simulink model "gm_rec_i2s"  (R2023b)
settings: Solver=VariableStepAuto  StartTime=0.0  StopTime=20  RelTol=1e-3
libraries: hdlsllib x2
(part 1 of 2)
settings Model: Creator=31651  LastModifiedBy=31651
settings DataIOCC: SignalLogging=off
settings OptimizationCC: BlockReduction=off  ConditionallyExecuteInputs=off  DefaultParameterBehavior=Inlined
settings DebuggingCC: AlgebraicLoopMsg=error  InheritedTsInSrcMsg=none
settings HardwareCC: ProdBitPerPointer=32  ProdBitPerSizeT=32  ProdBitPerPtrDiffT=32  ProdLargestAtomicFloat=None  ProdIntDivRoundTo=Undefined  ProdEndianess=Unspecified  ProdWordSize=32  ProdHWDeviceType=ASIC/FPGA->ASIC/FPGA  TargetBitPerPointer=64  TargetBitPerSizeT=64  TargetBitPerPtrDiffT=64  TargetLongLongMode=on  TargetIntDivRoundTo=Zero  TargetEndianess=LittleEndian  TargetWordSize=64  TargetHWDeviceType=Custom Processor->MATLAB Host Computer  ProdEqTarget=off

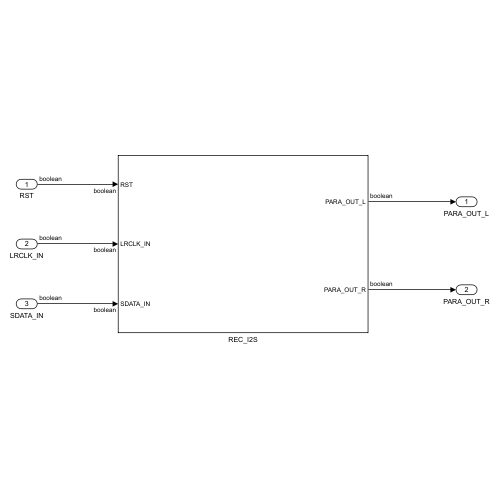
[thumbnail: Simulink's stored preview of the top-level diagram]
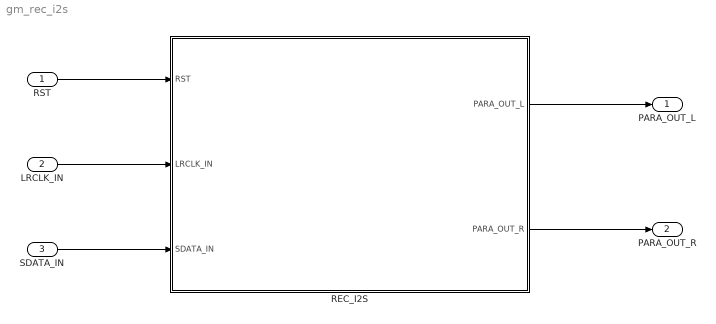
== system gm_rec_i2s ==
  RST : Inport  OutDataTypeStr=boolean  PortDimensions=1  SampleTime=1
  LRCLK_IN : Inport  Port=2  OutDataTypeStr=boolean  PortDimensions=1  SampleTime=1
  SDATA_IN : Inport  Port=3  OutDataTypeStr=boolean  PortDimensions=1  SampleTime=1
  REC_I2S : Subsystem
  PARA_OUT_L : Outport  SampleTime=1
  PARA_OUT_R : Outport  Port=2  SampleTime=1
  wires:
  RST/1 -> REC_I2S/1(RST)
  LRCLK_IN/1 -> REC_I2S/2(LRCLK_IN)
  SDATA_IN/1 -> REC_I2S/3(SDATA_IN)
  REC_I2S/1(PARA_OUT_L) -> PARA_OUT_L/1
  REC_I2S/2(PARA_OUT_R) -> PARA_OUT_R/1

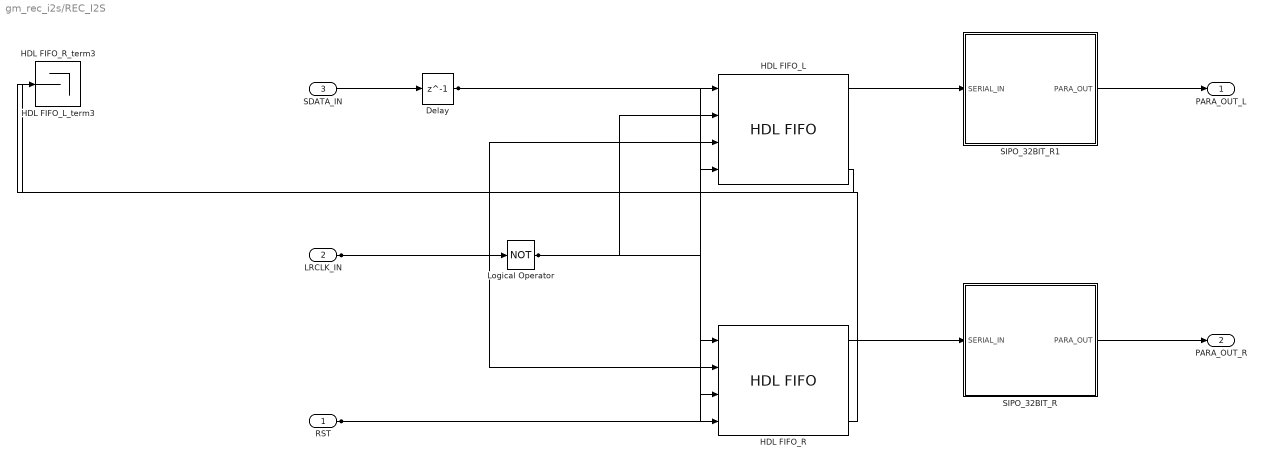
== system gm_rec_i2s/REC_I2S ==
  RST : Inport  OutDataTypeStr=boolean  PortDimensions=1  SampleTime=1
  LRCLK_IN : Inport  Port=2  OutDataTypeStr=boolean  PortDimensions=1  SampleTime=1
  SDATA_IN : Inport  Port=3  OutDataTypeStr=boolean  PortDimensions=1  SampleTime=1
  Delay : Delay  DelayLength=1  InitialCondition=0  SampleTime=1
  HDL FIFO_L : hdlsllib/HDL RAMs/HDL FIFO  fifo_size=32  mode=Classic  ratio=1  push_msg=Warning  pop_msg=Warning  show_empty=on  show_full=on  show_num=on  LabelModeActiveChoice_Mode=Classic  rst_port=on
  HDL FIFO_L_term3 : Terminator
  HDL FIFO_R : hdlsllib/HDL RAMs/HDL FIFO  fifo_size=32  mode=Classic  ratio=1  push_msg=Warning  pop_msg=Warning  show_empty=on  show_full=on  show_num=on  LabelModeActiveChoice_Mode=Classic  rst_port=on
  HDL FIFO_R_term3 : Terminator
  Logical Operator : Logic  Operator=NOT  AllPortsSameDT=off  OutDataTypeStr=boolean
  SIPO_32BIT_R : Subsystem
  SIPO_32BIT_R1 : Subsystem
  PARA_OUT_L : Outport  OutDataTypeStr=boolean  SampleTime=1
  PARA_OUT_R : Outport  Port=2  OutDataTypeStr=boolean  SampleTime=1
  wires:
  RST/1 -> HDL FIFO_R/4, HDL FIFO_L/4
  LRCLK_IN/1 -> Logical Operator/1, HDL FIFO_R/2, HDL FIFO_L/3
  SDATA_IN/1 -> Delay/1
  Delay/1 -> HDL FIFO_R/1, HDL FIFO_L/1
  HDL FIFO_L/1 -> SIPO_32BIT_R1/1(SERIAL_IN)
  HDL FIFO_L/4 -> HDL FIFO_L_term3/1
  HDL FIFO_R/1 -> SIPO_32BIT_R/1(SERIAL_IN)
  HDL FIFO_R/4 -> HDL FIFO_R_term3/1
  Logical Operator/1 -> HDL FIFO_R/3, HDL FIFO_L/2
  SIPO_32BIT_R/1(PARA_OUT) -> PARA_OUT_R/1
  SIPO_32BIT_R1/1(PARA_OUT) -> PARA_OUT_L/1

== system gm_rec_i2s/REC_I2S/SIPO_32BIT_R ==
  SERIAL_IN : Inport  OutDataTypeStr=boolean  PortDimensions=1  SampleTime=1
  Subsystem : Subsystem
  PARA_OUT : Outport  OutDataTypeStr=boolean  SampleTime=1  VectorParamsAs1DForOutWhenUnconnected=off
  wires:
  SERIAL_IN/1 -> Subsystem/1(SERIAL_IN)
  Subsystem/1(PARA_OUT_32BIT) -> PARA_OUT/1

== system gm_rec_i2s/REC_I2S/SIPO_32BIT_R1 ==
  SERIAL_IN : Inport  OutDataTypeStr=boolean  PortDimensions=1  SampleTime=1
  Subsystem : Subsystem
  PARA_OUT : Outport  OutDataTypeStr=boolean  SampleTime=1  VectorParamsAs1DForOutWhenUnconnected=off
  wires:
  SERIAL_IN/1 -> Subsystem/1(SERIAL_IN)
  Subsystem/1(PARA_OUT_32BIT) -> PARA_OUT/1

== system gm_rec_i2s/REC_I2S/SIPO_32BIT_R/Subsystem ==
  SERIAL_IN : Inport  OutDataTypeStr=boolean  PortDimensions=1  SampleTime=1
  SIPO_16BIT : Subsystem
  SIPO_16BIT1 : Subsystem
  Vector Concatenate : Concatenate
  PARA_OUT_32BIT : Outport  SampleTime=1
  wires:
  SERIAL_IN/1 -> SIPO_16BIT/1(SERIAL_IN)
  SIPO_16BIT/1(PARA_OUT) -> Vector Concatenate/2
  SIPO_16BIT/2(SERIAL_OUT) -> SIPO_16BIT1/1(SERIAL_IN)
  SIPO_16BIT1/1(PARA_OUT) -> Vector Concatenate/1
  Vector Concatenate/1 -> PARA_OUT_32BIT/1

== system gm_rec_i2s/REC_I2S/SIPO_32BIT_R1/Subsystem ==
  SERIAL_IN : Inport  OutDataTypeStr=boolean  PortDimensions=1  SampleTime=1
  SIPO_16BIT : Subsystem
  SIPO_16BIT1 : Subsystem
  Vector Concatenate : Concatenate
  PARA_OUT_32BIT : Outport  SampleTime=1
  wires:
  SERIAL_IN/1 -> SIPO_16BIT/1(SERIAL_IN)
  SIPO_16BIT/1(PARA_OUT) -> Vector Concatenate/2
  SIPO_16BIT/2(SERIAL_OUT) -> SIPO_16BIT1/1(SERIAL_IN)
  SIPO_16BIT1/1(PARA_OUT) -> Vector Concatenate/1
  Vector Concatenate/1 -> PARA_OUT_32BIT/1

== system gm_rec_i2s/REC_I2S/SIPO_32BIT_R/Subsystem/SIPO_16BIT ==
  SERIAL_IN : Inport  OutDataTypeStr=boolean  PortDimensions=1  SampleTime=1
  SIPO_8BIT : Subsystem
  SIPO_8BIT1 : Subsystem
  Vector Concatenate : Concatenate
  PARA_OUT : Outport  OutDataTypeStr=boolean  SampleTime=1  VectorParamsAs1DForOutWhenUnconnected=off
  SERIAL_OUT : Outport  Port=2  OutDataTypeStr=boolean  SampleTime=1  VectorParamsAs1DForOutWhenUnconnected=off
  wires:
  SERIAL_IN/1 -> SIPO_8BIT/1(SERIAL_IN)
  SIPO_8BIT/1(PARA_OUT) -> Vector Concatenate/2
  SIPO_8BIT/2(SERIAL_OUT) -> SIPO_8BIT1/1(SERIAL_IN)
  SIPO_8BIT1/1(PARA_OUT) -> Vector Concatenate/1
  SIPO_8BIT1/2(SERIAL_OUT) -> SERIAL_OUT/1
  Vector Concatenate/1 -> PARA_OUT/1

== system gm_rec_i2s/REC_I2S/SIPO_32BIT_R/Subsystem/SIPO_16BIT1 ==
  SERIAL_IN : Inport  OutDataTypeStr=boolean  PortDimensions=1  SampleTime=1
  SIPO_8BIT : Subsystem
  SIPO_8BIT1 : Subsystem
  Vector Concatenate : Concatenate
  PARA_OUT : Outport  OutDataTypeStr=boolean  SampleTime=1  VectorParamsAs1DForOutWhenUnconnected=off
  wires:
  SERIAL_IN/1 -> SIPO_8BIT/1(SERIAL_IN)
  SIPO_8BIT/1(PARA_OUT) -> Vector Concatenate/2
  SIPO_8BIT/2(SERIAL_OUT) -> SIPO_8BIT1/1(SERIAL_IN)
  SIPO_8BIT1/1(PARA_OUT) -> Vector Concatenate/1
  Vector Concatenate/1 -> PARA_OUT/1

== system gm_rec_i2s/REC_I2S/SIPO_32BIT_R1/Subsystem/SIPO_16BIT ==
  SERIAL_IN : Inport  OutDataTypeStr=boolean  PortDimensions=1  SampleTime=1
  SIPO_8BIT : Subsystem
  SIPO_8BIT1 : Subsystem
  Vector Concatenate : Concatenate
  PARA_OUT : Outport  OutDataTypeStr=boolean  SampleTime=1  VectorParamsAs1DForOutWhenUnconnected=off
  SERIAL_OUT : Outport  Port=2  OutDataTypeStr=boolean  SampleTime=1  VectorParamsAs1DForOutWhenUnconnected=off
  wires:
  SERIAL_IN/1 -> SIPO_8BIT/1(SERIAL_IN)
  SIPO_8BIT/1(PARA_OUT) -> Vector Concatenate/2
  SIPO_8BIT/2(SERIAL_OUT) -> SIPO_8BIT1/1(SERIAL_IN)
  SIPO_8BIT1/1(PARA_OUT) -> Vector Concatenate/1
  SIPO_8BIT1/2(SERIAL_OUT) -> SERIAL_OUT/1
  Vector Concatenate/1 -> PARA_OUT/1

== system gm_rec_i2s/REC_I2S/SIPO_32BIT_R1/Subsystem/SIPO_16BIT1 ==
  SERIAL_IN : Inport  OutDataTypeStr=boolean  PortDimensions=1  SampleTime=1
  SIPO_8BIT : Subsystem
  SIPO_8BIT1 : Subsystem
  Vector Concatenate : Concatenate
  PARA_OUT : Outport  OutDataTypeStr=boolean  SampleTime=1  VectorParamsAs1DForOutWhenUnconnected=off
  wires:
  SERIAL_IN/1 -> SIPO_8BIT/1(SERIAL_IN)
  SIPO_8BIT/1(PARA_OUT) -> Vector Concatenate/2
  SIPO_8BIT/2(SERIAL_OUT) -> SIPO_8BIT1/1(SERIAL_IN)
  SIPO_8BIT1/1(PARA_OUT) -> Vector Concatenate/1
  Vector Concatenate/1 -> PARA_OUT/1

== system gm_rec_i2s/REC_I2S/SIPO_32BIT_R/Subsystem/SIPO_16BIT/SIPO_8BIT ==
  SERIAL_IN : Inport  OutDataTypeStr=boolean  PortDimensions=1  SampleTime=1
  SIPO_4BIT : Subsystem
  SIPO_4BIT1 : Subsystem
  Vector Concatenate : Concatenate
  PARA_OUT : Outport  SampleTime=1  VectorParamsAs1DForOutWhenUnconnected=off
  SERIAL_OUT : Outport  Port=2  SampleTime=1  VectorParamsAs1DForOutWhenUnconnected=off
  wires:
  SERIAL_IN/1 -> SIPO_4BIT/1(SERIAL_IN)
  SIPO_4BIT/1(PARA_OUT) -> Vector Concatenate/2
  SIPO_4BIT/2(SERIAL_OUT) -> SIPO_4BIT1/1(SERIAL_IN)
  SIPO_4BIT1/1(PARA_OUT) -> Vector Concatenate/1
  SIPO_4BIT1/2(SERIAL_OUT) -> SERIAL_OUT/1
  Vector Concatenate/1 -> PARA_OUT/1

== system gm_rec_i2s/REC_I2S/SIPO_32BIT_R/Subsystem/SIPO_16BIT/SIPO_8BIT1 ==
  SERIAL_IN : Inport  OutDataTypeStr=boolean  PortDimensions=1  SampleTime=1
  SIPO_4BIT : Subsystem
  SIPO_4BIT1 : Subsystem
  Vector Concatenate : Concatenate
  PARA_OUT : Outport  SampleTime=1  VectorParamsAs1DForOutWhenUnconnected=off
  SERIAL_OUT : Outport  Port=2  SampleTime=1  VectorParamsAs1DForOutWhenUnconnected=off
  wires:
  SERIAL_IN/1 -> SIPO_4BIT/1(SERIAL_IN)
  SIPO_4BIT/1(PARA_OUT) -> Vector Concatenate/2
  SIPO_4BIT/2(SERIAL_OUT) -> SIPO_4BIT1/1(SERIAL_IN)
  SIPO_4BIT1/1(PARA_OUT) -> Vector Concatenate/1
  SIPO_4BIT1/2(SERIAL_OUT) -> SERIAL_OUT/1
  Vector Concatenate/1 -> PARA_OUT/1

== system gm_rec_i2s/REC_I2S/SIPO_32BIT_R/Subsystem/SIPO_16BIT1/SIPO_8BIT ==
  SERIAL_IN : Inport  OutDataTypeStr=boolean  PortDimensions=1  SampleTime=1
  SIPO_4BIT : Subsystem
  SIPO_4BIT1 : Subsystem
  Vector Concatenate : Concatenate
  PARA_OUT : Outport  SampleTime=1  VectorParamsAs1DForOutWhenUnconnected=off
  SERIAL_OUT : Outport  Port=2  SampleTime=1  VectorParamsAs1DForOutWhenUnconnected=off
  wires:
  SERIAL_IN/1 -> SIPO_4BIT/1(SERIAL_IN)
  SIPO_4BIT/1(PARA_OUT) -> Vector Concatenate/2
  SIPO_4BIT/2(SERIAL_OUT) -> SIPO_4BIT1/1(SERIAL_IN)
  SIPO_4BIT1/1(PARA_OUT) -> Vector Concatenate/1
  SIPO_4BIT1/2(SERIAL_OUT) -> SERIAL_OUT/1
  Vector Concatenate/1 -> PARA_OUT/1

== system gm_rec_i2s/REC_I2S/SIPO_32BIT_R/Subsystem/SIPO_16BIT1/SIPO_8BIT1 ==
  SERIAL_IN : Inport  OutDataTypeStr=boolean  PortDimensions=1  SampleTime=1
  SIPO_4BIT : Subsystem
  SIPO_4BIT1 : Subsystem
  Vector Concatenate : Concatenate
  PARA_OUT : Outport  SampleTime=1  VectorParamsAs1DForOutWhenUnconnected=off
  wires:
  SERIAL_IN/1 -> SIPO_4BIT/1(SERIAL_IN)
  SIPO_4BIT/1(PARA_OUT) -> Vector Concatenate/2
  SIPO_4BIT/2(SERIAL_OUT) -> SIPO_4BIT1/1(SERIAL_IN)
  SIPO_4BIT1/1(PARA_OUT) -> Vector Concatenate/1
  Vector Concatenate/1 -> PARA_OUT/1

== system gm_rec_i2s/REC_I2S/SIPO_32BIT_R1/Subsystem/SIPO_16BIT/SIPO_8BIT ==
  SERIAL_IN : Inport  OutDataTypeStr=boolean  PortDimensions=1  SampleTime=1
  SIPO_4BIT : Subsystem
  SIPO_4BIT1 : Subsystem
  Vector Concatenate : Concatenate
  PARA_OUT : Outport  SampleTime=1  VectorParamsAs1DForOutWhenUnconnected=off
  SERIAL_OUT : Outport  Port=2  SampleTime=1  VectorParamsAs1DForOutWhenUnconnected=off
  wires:
  SERIAL_IN/1 -> SIPO_4BIT/1(SERIAL_IN)
  SIPO_4BIT/1(PARA_OUT) -> Vector Concatenate/2
  SIPO_4BIT/2(SERIAL_OUT) -> SIPO_4BIT1/1(SERIAL_IN)
  SIPO_4BIT1/1(PARA_OUT) -> Vector Concatenate/1
  SIPO_4BIT1/2(SERIAL_OUT) -> SERIAL_OUT/1
  Vector Concatenate/1 -> PARA_OUT/1

== system gm_rec_i2s/REC_I2S/SIPO_32BIT_R1/Subsystem/SIPO_16BIT/SIPO_8BIT1 ==
  SERIAL_IN : Inport  OutDataTypeStr=boolean  PortDimensions=1  SampleTime=1
  SIPO_4BIT : Subsystem
  SIPO_4BIT1 : Subsystem
  Vector Concatenate : Concatenate
  PARA_OUT : Outport  SampleTime=1  VectorParamsAs1DForOutWhenUnconnected=off
  SERIAL_OUT : Outport  Port=2  SampleTime=1  VectorParamsAs1DForOutWhenUnconnected=off
  wires:
  SERIAL_IN/1 -> SIPO_4BIT/1(SERIAL_IN)
  SIPO_4BIT/1(PARA_OUT) -> Vector Concatenate/2
  SIPO_4BIT/2(SERIAL_OUT) -> SIPO_4BIT1/1(SERIAL_IN)
  SIPO_4BIT1/1(PARA_OUT) -> Vector Concatenate/1
  SIPO_4BIT1/2(SERIAL_OUT) -> SERIAL_OUT/1
  Vector Concatenate/1 -> PARA_OUT/1

== system gm_rec_i2s/REC_I2S/SIPO_32BIT_R1/Subsystem/SIPO_16BIT1/SIPO_8BIT ==
  SERIAL_IN : Inport  OutDataTypeStr=boolean  PortDimensions=1  SampleTime=1
  SIPO_4BIT : Subsystem
  SIPO_4BIT1 : Subsystem
  Vector Concatenate : Concatenate
  PARA_OUT : Outport  SampleTime=1  VectorParamsAs1DForOutWhenUnconnected=off
  SERIAL_OUT : Outport  Port=2  SampleTime=1  VectorParamsAs1DForOutWhenUnconnected=off
  wires:
  SERIAL_IN/1 -> SIPO_4BIT/1(SERIAL_IN)
  SIPO_4BIT/1(PARA_OUT) -> Vector Concatenate/2
  SIPO_4BIT/2(SERIAL_OUT) -> SIPO_4BIT1/1(SERIAL_IN)
  SIPO_4BIT1/1(PARA_OUT) -> Vector Concatenate/1
  SIPO_4BIT1/2(SERIAL_OUT) -> SERIAL_OUT/1
  Vector Concatenate/1 -> PARA_OUT/1

== system gm_rec_i2s/REC_I2S/SIPO_32BIT_R1/Subsystem/SIPO_16BIT1/SIPO_8BIT1 ==
  SERIAL_IN : Inport  OutDataTypeStr=boolean  PortDimensions=1  SampleTime=1
  SIPO_4BIT : Subsystem
  SIPO_4BIT1 : Subsystem
  Vector Concatenate : Concatenate
  PARA_OUT : Outport  SampleTime=1  VectorParamsAs1DForOutWhenUnconnected=off
  wires:
  SERIAL_IN/1 -> SIPO_4BIT/1(SERIAL_IN)
  SIPO_4BIT/1(PARA_OUT) -> Vector Concatenate/2
  SIPO_4BIT/2(SERIAL_OUT) -> SIPO_4BIT1/1(SERIAL_IN)
  SIPO_4BIT1/1(PARA_OUT) -> Vector Concatenate/1
  Vector Concatenate/1 -> PARA_OUT/1

== system gm_rec_i2s/REC_I2S/SIPO_32BIT_R/Subsystem/SIPO_16BIT/SIPO_8BIT/SIPO_4BIT ==
  SERIAL_IN : Inport  OutDataTypeStr=boolean  PortDimensions=1  SampleTime=1
  2BIT_SIPO : Subsystem
  2BIT_SIPO1 : Subsystem
  Vector Concatenate : Concatenate
  PARA_OUT : Outport  SampleTime=1  VectorParamsAs1DForOutWhenUnconnected=off
  SERIAL_OUT : Outport  Port=2  SampleTime=1  VectorParamsAs1DForOutWhenUnconnected=off
  wires:
  SERIAL_IN/1 -> 2BIT_SIPO/1(SERIAL_IN)
  2BIT_SIPO/1(PARA_OUT) -> Vector Concatenate/2
  2BIT_SIPO/2(SERIAL_OUT) -> 2BIT_SIPO1/1(SERIAL_IN)
  2BIT_SIPO1/1(PARA_OUT) -> Vector Concatenate/1
  2BIT_SIPO1/2(SERIAL_OUT) -> SERIAL_OUT/1
  Vector Concatenate/1 -> PARA_OUT/1

== system gm_rec_i2s/REC_I2S/SIPO_32BIT_R/Subsystem/SIPO_16BIT/SIPO_8BIT/SIPO_4BIT1 ==
  SERIAL_IN : Inport  OutDataTypeStr=boolean  PortDimensions=1  SampleTime=1
  2BIT_SIPO : Subsystem
  2BIT_SIPO1 : Subsystem
  Vector Concatenate : Concatenate
  PARA_OUT : Outport  SampleTime=1  VectorParamsAs1DForOutWhenUnconnected=off
  SERIAL_OUT : Outport  Port=2  SampleTime=1  VectorParamsAs1DForOutWhenUnconnected=off
  wires:
  SERIAL_IN/1 -> 2BIT_SIPO/1(SERIAL_IN)
  2BIT_SIPO/1(PARA_OUT) -> Vector Concatenate/2
  2BIT_SIPO/2(SERIAL_OUT) -> 2BIT_SIPO1/1(SERIAL_IN)
  2BIT_SIPO1/1(PARA_OUT) -> Vector Concatenate/1
  2BIT_SIPO1/2(SERIAL_OUT) -> SERIAL_OUT/1
  Vector Concatenate/1 -> PARA_OUT/1

== system gm_rec_i2s/REC_I2S/SIPO_32BIT_R/Subsystem/SIPO_16BIT/SIPO_8BIT1/SIPO_4BIT ==
  SERIAL_IN : Inport  OutDataTypeStr=boolean  PortDimensions=1  SampleTime=1
  2BIT_SIPO : Subsystem
  2BIT_SIPO1 : Subsystem
  Vector Concatenate : Concatenate
  PARA_OUT : Outport  SampleTime=1  VectorParamsAs1DForOutWhenUnconnected=off
  SERIAL_OUT : Outport  Port=2  SampleTime=1  VectorParamsAs1DForOutWhenUnconnected=off
  wires:
  SERIAL_IN/1 -> 2BIT_SIPO/1(SERIAL_IN)
  2BIT_SIPO/1(PARA_OUT) -> Vector Concatenate/2
  2BIT_SIPO/2(SERIAL_OUT) -> 2BIT_SIPO1/1(SERIAL_IN)
  2BIT_SIPO1/1(PARA_OUT) -> Vector Concatenate/1
  2BIT_SIPO1/2(SERIAL_OUT) -> SERIAL_OUT/1
  Vector Concatenate/1 -> PARA_OUT/1

== system gm_rec_i2s/REC_I2S/SIPO_32BIT_R/Subsystem/SIPO_16BIT/SIPO_8BIT1/SIPO_4BIT1 ==
  SERIAL_IN : Inport  OutDataTypeStr=boolean  PortDimensions=1  SampleTime=1
  2BIT_SIPO : Subsystem
  2BIT_SIPO1 : Subsystem
  Vector Concatenate : Concatenate
  PARA_OUT : Outport  SampleTime=1  VectorParamsAs1DForOutWhenUnconnected=off
  SERIAL_OUT : Outport  Port=2  SampleTime=1  VectorParamsAs1DForOutWhenUnconnected=off
  wires:
  SERIAL_IN/1 -> 2BIT_SIPO/1(SERIAL_IN)
  2BIT_SIPO/1(PARA_OUT) -> Vector Concatenate/2
  2BIT_SIPO/2(SERIAL_OUT) -> 2BIT_SIPO1/1(SERIAL_IN)
  2BIT_SIPO1/1(PARA_OUT) -> Vector Concatenate/1
  2BIT_SIPO1/2(SERIAL_OUT) -> SERIAL_OUT/1
  Vector Concatenate/1 -> PARA_OUT/1

== system gm_rec_i2s/REC_I2S/SIPO_32BIT_R/Subsystem/SIPO_16BIT1/SIPO_8BIT/SIPO_4BIT ==
  SERIAL_IN : Inport  OutDataTypeStr=boolean  PortDimensions=1  SampleTime=1
  2BIT_SIPO : Subsystem
  2BIT_SIPO1 : Subsystem
  Vector Concatenate : Concatenate
  PARA_OUT : Outport  SampleTime=1  VectorParamsAs1DForOutWhenUnconnected=off
  SERIAL_OUT : Outport  Port=2  SampleTime=1  VectorParamsAs1DForOutWhenUnconnected=off
  wires:
  SERIAL_IN/1 -> 2BIT_SIPO/1(SERIAL_IN)
  2BIT_SIPO/1(PARA_OUT) -> Vector Concatenate/2
  2BIT_SIPO/2(SERIAL_OUT) -> 2BIT_SIPO1/1(SERIAL_IN)
  2BIT_SIPO1/1(PARA_OUT) -> Vector Concatenate/1
  2BIT_SIPO1/2(SERIAL_OUT) -> SERIAL_OUT/1
  Vector Concatenate/1 -> PARA_OUT/1

== system gm_rec_i2s/REC_I2S/SIPO_32BIT_R/Subsystem/SIPO_16BIT1/SIPO_8BIT/SIPO_4BIT1 ==
  SERIAL_IN : Inport  OutDataTypeStr=boolean  PortDimensions=1  SampleTime=1
  2BIT_SIPO : Subsystem
  2BIT_SIPO1 : Subsystem
  Vector Concatenate : Concatenate
  PARA_OUT : Outport  SampleTime=1  VectorParamsAs1DForOutWhenUnconnected=off
  SERIAL_OUT : Outport  Port=2  SampleTime=1  VectorParamsAs1DForOutWhenUnconnected=off
  wires:
  SERIAL_IN/1 -> 2BIT_SIPO/1(SERIAL_IN)
  2BIT_SIPO/1(PARA_OUT) -> Vector Concatenate/2
  2BIT_SIPO/2(SERIAL_OUT) -> 2BIT_SIPO1/1(SERIAL_IN)
  2BIT_SIPO1/1(PARA_OUT) -> Vector Concatenate/1
  2BIT_SIPO1/2(SERIAL_OUT) -> SERIAL_OUT/1
  Vector Concatenate/1 -> PARA_OUT/1

== system gm_rec_i2s/REC_I2S/SIPO_32BIT_R/Subsystem/SIPO_16BIT1/SIPO_8BIT1/SIPO_4BIT ==
  SERIAL_IN : Inport  OutDataTypeStr=boolean  PortDimensions=1  SampleTime=1
  2BIT_SIPO : Subsystem
  2BIT_SIPO1 : Subsystem
  Vector Concatenate : Concatenate
  PARA_OUT : Outport  SampleTime=1  VectorParamsAs1DForOutWhenUnconnected=off
  SERIAL_OUT : Outport  Port=2  SampleTime=1  VectorParamsAs1DForOutWhenUnconnected=off
  wires:
  SERIAL_IN/1 -> 2BIT_SIPO/1(SERIAL_IN)
  2BIT_SIPO/1(PARA_OUT) -> Vector Concatenate/2
  2BIT_SIPO/2(SERIAL_OUT) -> 2BIT_SIPO1/1(SERIAL_IN)
  2BIT_SIPO1/1(PARA_OUT) -> Vector Concatenate/1
  2BIT_SIPO1/2(SERIAL_OUT) -> SERIAL_OUT/1
  Vector Concatenate/1 -> PARA_OUT/1

== system gm_rec_i2s/REC_I2S/SIPO_32BIT_R/Subsystem/SIPO_16BIT1/SIPO_8BIT1/SIPO_4BIT1 ==
  SERIAL_IN : Inport  OutDataTypeStr=boolean  PortDimensions=1  SampleTime=1
  2BIT_SIPO : Subsystem
  2BIT_SIPO1 : Subsystem
  Vector Concatenate : Concatenate
  PARA_OUT : Outport  SampleTime=1  VectorParamsAs1DForOutWhenUnconnected=off
  wires:
  SERIAL_IN/1 -> 2BIT_SIPO/1(SERIAL_IN)
  2BIT_SIPO/1(PARA_OUT) -> Vector Concatenate/2
  2BIT_SIPO/2(SERIAL_OUT) -> 2BIT_SIPO1/1(SERIAL_IN)
  2BIT_SIPO1/1(PARA_OUT) -> Vector Concatenate/1
  Vector Concatenate/1 -> PARA_OUT/1

== system gm_rec_i2s/REC_I2S/SIPO_32BIT_R1/Subsystem/SIPO_16BIT/SIPO_8BIT/SIPO_4BIT ==
  SERIAL_IN : Inport  OutDataTypeStr=boolean  PortDimensions=1  SampleTime=1
  2BIT_SIPO : Subsystem
  2BIT_SIPO1 : Subsystem
  Vector Concatenate : Concatenate
  PARA_OUT : Outport  SampleTime=1  VectorParamsAs1DForOutWhenUnconnected=off
  SERIAL_OUT : Outport  Port=2  SampleTime=1  VectorParamsAs1DForOutWhenUnconnected=off
  wires:
  SERIAL_IN/1 -> 2BIT_SIPO/1(SERIAL_IN)
  2BIT_SIPO/1(PARA_OUT) -> Vector Concatenate/2
  2BIT_SIPO/2(SERIAL_OUT) -> 2BIT_SIPO1/1(SERIAL_IN)
  2BIT_SIPO1/1(PARA_OUT) -> Vector Concatenate/1
  2BIT_SIPO1/2(SERIAL_OUT) -> SERIAL_OUT/1
  Vector Concatenate/1 -> PARA_OUT/1

== system gm_rec_i2s/REC_I2S/SIPO_32BIT_R1/Subsystem/SIPO_16BIT/SIPO_8BIT/SIPO_4BIT1 ==
  SERIAL_IN : Inport  OutDataTypeStr=boolean  PortDimensions=1  SampleTime=1
  2BIT_SIPO : Subsystem
  2BIT_SIPO1 : Subsystem
  Vector Concatenate : Concatenate
  PARA_OUT : Outport  SampleTime=1  VectorParamsAs1DForOutWhenUnconnected=off
  SERIAL_OUT : Outport  Port=2  SampleTime=1  VectorParamsAs1DForOutWhenUnconnected=off
  wires:
  SERIAL_IN/1 -> 2BIT_SIPO/1(SERIAL_IN)
  2BIT_SIPO/1(PARA_OUT) -> Vector Concatenate/2
  2BIT_SIPO/2(SERIAL_OUT) -> 2BIT_SIPO1/1(SERIAL_IN)
  2BIT_SIPO1/1(PARA_OUT) -> Vector Concatenate/1
  2BIT_SIPO1/2(SERIAL_OUT) -> SERIAL_OUT/1
  Vector Concatenate/1 -> PARA_OUT/1

== system gm_rec_i2s/REC_I2S/SIPO_32BIT_R1/Subsystem/SIPO_16BIT/SIPO_8BIT1/SIPO_4BIT ==
  SERIAL_IN : Inport  OutDataTypeStr=boolean  PortDimensions=1  SampleTime=1
  2BIT_SIPO : Subsystem
  2BIT_SIPO1 : Subsystem
  Vector Concatenate : Concatenate
  PARA_OUT : Outport  SampleTime=1  VectorParamsAs1DForOutWhenUnconnected=off
  SERIAL_OUT : Outport  Port=2  SampleTime=1  VectorParamsAs1DForOutWhenUnconnected=off
  wires:
  SERIAL_IN/1 -> 2BIT_SIPO/1(SERIAL_IN)
  2BIT_SIPO/1(PARA_OUT) -> Vector Concatenate/2
  2BIT_SIPO/2(SERIAL_OUT) -> 2BIT_SIPO1/1(SERIAL_IN)
  2BIT_SIPO1/1(PARA_OUT) -> Vector Concatenate/1
  2BIT_SIPO1/2(SERIAL_OUT) -> SERIAL_OUT/1
  Vector Concatenate/1 -> PARA_OUT/1

== system gm_rec_i2s/REC_I2S/SIPO_32BIT_R1/Subsystem/SIPO_16BIT/SIPO_8BIT1/SIPO_4BIT1 ==
  SERIAL_IN : Inport  OutDataTypeStr=boolean  PortDimensions=1  SampleTime=1
  2BIT_SIPO : Subsystem
  2BIT_SIPO1 : Subsystem
  Vector Concatenate : Concatenate
  PARA_OUT : Outport  SampleTime=1  VectorParamsAs1DForOutWhenUnconnected=off
  SERIAL_OUT : Outport  Port=2  SampleTime=1  VectorParamsAs1DForOutWhenUnconnected=off
  wires:
  SERIAL_IN/1 -> 2BIT_SIPO/1(SERIAL_IN)
  2BIT_SIPO/1(PARA_OUT) -> Vector Concatenate/2
  2BIT_SIPO/2(SERIAL_OUT) -> 2BIT_SIPO1/1(SERIAL_IN)
  2BIT_SIPO1/1(PARA_OUT) -> Vector Concatenate/1
  2BIT_SIPO1/2(SERIAL_OUT) -> SERIAL_OUT/1
  Vector Concatenate/1 -> PARA_OUT/1

== system gm_rec_i2s/REC_I2S/SIPO_32BIT_R1/Subsystem/SIPO_16BIT1/SIPO_8BIT/SIPO_4BIT ==
  SERIAL_IN : Inport  OutDataTypeStr=boolean  PortDimensions=1  SampleTime=1
  2BIT_SIPO : Subsystem
  2BIT_SIPO1 : Subsystem
  Vector Concatenate : Concatenate
  PARA_OUT : Outport  SampleTime=1  VectorParamsAs1DForOutWhenUnconnected=off
  SERIAL_OUT : Outport  Port=2  SampleTime=1  VectorParamsAs1DForOutWhenUnconnected=off
  wires:
  SERIAL_IN/1 -> 2BIT_SIPO/1(SERIAL_IN)
  2BIT_SIPO/1(PARA_OUT) -> Vector Concatenate/2
  2BIT_SIPO/2(SERIAL_OUT) -> 2BIT_SIPO1/1(SERIAL_IN)
  2BIT_SIPO1/1(PARA_OUT) -> Vector Concatenate/1
  2BIT_SIPO1/2(SERIAL_OUT) -> SERIAL_OUT/1
  Vector Concatenate/1 -> PARA_OUT/1

== system gm_rec_i2s/REC_I2S/SIPO_32BIT_R1/Subsystem/SIPO_16BIT1/SIPO_8BIT/SIPO_4BIT1 ==
  SERIAL_IN : Inport  OutDataTypeStr=boolean  PortDimensions=1  SampleTime=1
  2BIT_SIPO : Subsystem
  2BIT_SIPO1 : Subsystem
  Vector Concatenate : Concatenate
  PARA_OUT : Outport  SampleTime=1  VectorParamsAs1DForOutWhenUnconnected=off
  SERIAL_OUT : Outport  Port=2  SampleTime=1  VectorParamsAs1DForOutWhenUnconnected=off
  wires:
  SERIAL_IN/1 -> 2BIT_SIPO/1(SERIAL_IN)
  2BIT_SIPO/1(PARA_OUT) -> Vector Concatenate/2
  2BIT_SIPO/2(SERIAL_OUT) -> 2BIT_SIPO1/1(SERIAL_IN)
  2BIT_SIPO1/1(PARA_OUT) -> Vector Concatenate/1
  2BIT_SIPO1/2(SERIAL_OUT) -> SERIAL_OUT/1
  Vector Concatenate/1 -> PARA_OUT/1

== system gm_rec_i2s/REC_I2S/SIPO_32BIT_R1/Subsystem/SIPO_16BIT1/SIPO_8BIT1/SIPO_4BIT ==
  SERIAL_IN : Inport  OutDataTypeStr=boolean  PortDimensions=1  SampleTime=1
  2BIT_SIPO : Subsystem
  2BIT_SIPO1 : Subsystem
  Vector Concatenate : Concatenate
  PARA_OUT : Outport  SampleTime=1  VectorParamsAs1DForOutWhenUnconnected=off
  SERIAL_OUT : Outport  Port=2  SampleTime=1  VectorParamsAs1DForOutWhenUnconnected=off
  wires:
  SERIAL_IN/1 -> 2BIT_SIPO/1(SERIAL_IN)
  2BIT_SIPO/1(PARA_OUT) -> Vector Concatenate/2
  2BIT_SIPO/2(SERIAL_OUT) -> 2BIT_SIPO1/1(SERIAL_IN)
  2BIT_SIPO1/1(PARA_OUT) -> Vector Concatenate/1
  2BIT_SIPO1/2(SERIAL_OUT) -> SERIAL_OUT/1
  Vector Concatenate/1 -> PARA_OUT/1

== system gm_rec_i2s/REC_I2S/SIPO_32BIT_R1/Subsystem/SIPO_16BIT1/SIPO_8BIT1/SIPO_4BIT1 ==
  SERIAL_IN : Inport  OutDataTypeStr=boolean  PortDimensions=1  SampleTime=1
  2BIT_SIPO : Subsystem
  2BIT_SIPO1 : Subsystem
  Vector Concatenate : Concatenate
  PARA_OUT : Outport  SampleTime=1  VectorParamsAs1DForOutWhenUnconnected=off
  wires:
  SERIAL_IN/1 -> 2BIT_SIPO/1(SERIAL_IN)
  2BIT_SIPO/1(PARA_OUT) -> Vector Concatenate/2
  2BIT_SIPO/2(SERIAL_OUT) -> 2BIT_SIPO1/1(SERIAL_IN)
  2BIT_SIPO1/1(PARA_OUT) -> Vector Concatenate/1
  Vector Concatenate/1 -> PARA_OUT/1

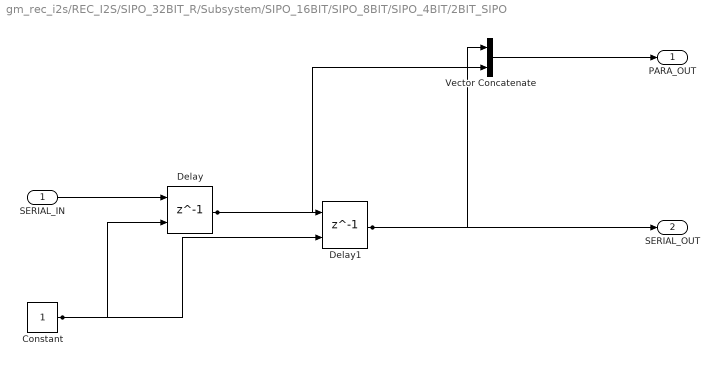
== system gm_rec_i2s/REC_I2S/SIPO_32BIT_R/Subsystem/SIPO_16BIT/SIPO_8BIT/SIPO_4BIT/2BIT_SIPO ==
  SERIAL_IN : Inport  OutDataTypeStr=boolean  PortDimensions=1  SampleTime=1
  Constant : Constant  OutDataTypeStr=boolean  SampleTime=1
  Delay : Delay  DelayLength=1  InitialCondition=0  ShowEnablePort=on  SampleTime=1
      settings: InputPortMap=u0,e6
  Delay1 : Delay  DelayLength=1  InitialCondition=0  ShowEnablePort=on  SampleTime=1
      settings: InputPortMap=u0,e6
  Vector Concatenate : Concatenate
  PARA_OUT : Outport  SampleTime=1  VectorParamsAs1DForOutWhenUnconnected=off
  SERIAL_OUT : Outport  Port=2  SampleTime=1  VectorParamsAs1DForOutWhenUnconnected=off
  wires:
  SERIAL_IN/1 -> Delay/1
  Constant/1 -> Delay1/2, Delay/2
  Delay/1 -> Vector Concatenate/2, Delay1/1
  Delay1/1 -> Vector Concatenate/1, SERIAL_OUT/1
  Vector Concatenate/1 -> PARA_OUT/1

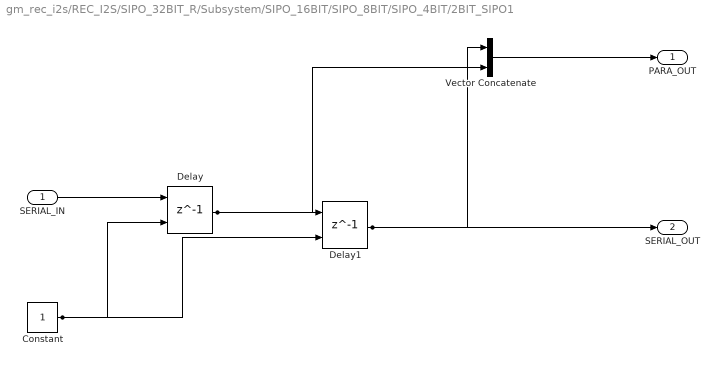
== system gm_rec_i2s/REC_I2S/SIPO_32BIT_R/Subsystem/SIPO_16BIT/SIPO_8BIT/SIPO_4BIT/2BIT_SIPO1 ==
  SERIAL_IN : Inport  OutDataTypeStr=boolean  PortDimensions=1  SampleTime=1
  Constant : Constant  OutDataTypeStr=boolean  SampleTime=1
  Delay : Delay  DelayLength=1  InitialCondition=0  ShowEnablePort=on  SampleTime=1
      settings: InputPortMap=u0,e6
  Delay1 : Delay  DelayLength=1  InitialCondition=0  ShowEnablePort=on  SampleTime=1
      settings: InputPortMap=u0,e6
  Vector Concatenate : Concatenate
  PARA_OUT : Outport  SampleTime=1  VectorParamsAs1DForOutWhenUnconnected=off
  SERIAL_OUT : Outport  Port=2  SampleTime=1  VectorParamsAs1DForOutWhenUnconnected=off
  wires:
  SERIAL_IN/1 -> Delay/1
  Constant/1 -> Delay1/2, Delay/2
  Delay/1 -> Vector Concatenate/2, Delay1/1
  Delay1/1 -> Vector Concatenate/1, SERIAL_OUT/1
  Vector Concatenate/1 -> PARA_OUT/1

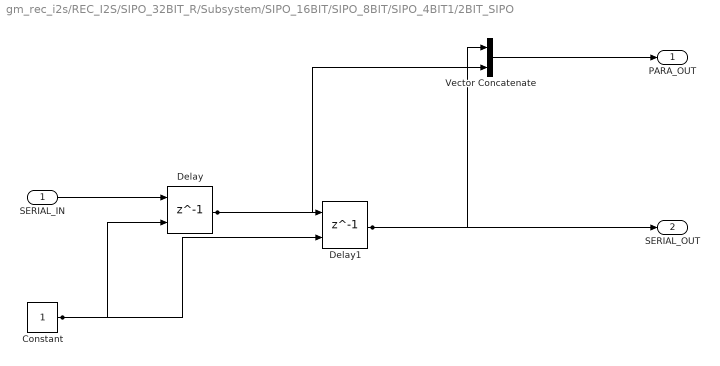
== system gm_rec_i2s/REC_I2S/SIPO_32BIT_R/Subsystem/SIPO_16BIT/SIPO_8BIT/SIPO_4BIT1/2BIT_SIPO ==
  SERIAL_IN : Inport  OutDataTypeStr=boolean  PortDimensions=1  SampleTime=1
  Constant : Constant  OutDataTypeStr=boolean  SampleTime=1
  Delay : Delay  DelayLength=1  InitialCondition=0  ShowEnablePort=on  SampleTime=1
      settings: InputPortMap=u0,e6
  Delay1 : Delay  DelayLength=1  InitialCondition=0  ShowEnablePort=on  SampleTime=1
      settings: InputPortMap=u0,e6
  Vector Concatenate : Concatenate
  PARA_OUT : Outport  SampleTime=1  VectorParamsAs1DForOutWhenUnconnected=off
  SERIAL_OUT : Outport  Port=2  SampleTime=1  VectorParamsAs1DForOutWhenUnconnected=off
  wires:
  SERIAL_IN/1 -> Delay/1
  Constant/1 -> Delay1/2, Delay/2
  Delay/1 -> Vector Concatenate/2, Delay1/1
  Delay1/1 -> Vector Concatenate/1, SERIAL_OUT/1
  Vector Concatenate/1 -> PARA_OUT/1

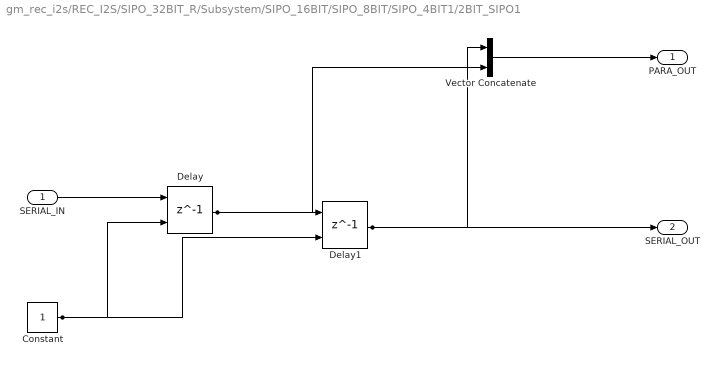
== system gm_rec_i2s/REC_I2S/SIPO_32BIT_R/Subsystem/SIPO_16BIT/SIPO_8BIT/SIPO_4BIT1/2BIT_SIPO1 ==
  SERIAL_IN : Inport  OutDataTypeStr=boolean  PortDimensions=1  SampleTime=1
  Constant : Constant  OutDataTypeStr=boolean  SampleTime=1
  Delay : Delay  DelayLength=1  InitialCondition=0  ShowEnablePort=on  SampleTime=1
      settings: InputPortMap=u0,e6
  Delay1 : Delay  DelayLength=1  InitialCondition=0  ShowEnablePort=on  SampleTime=1
      settings: InputPortMap=u0,e6
  Vector Concatenate : Concatenate
  PARA_OUT : Outport  SampleTime=1  VectorParamsAs1DForOutWhenUnconnected=off
  SERIAL_OUT : Outport  Port=2  SampleTime=1  VectorParamsAs1DForOutWhenUnconnected=off
  wires:
  SERIAL_IN/1 -> Delay/1
  Constant/1 -> Delay1/2, Delay/2
  Delay/1 -> Vector Concatenate/2, Delay1/1
  Delay1/1 -> Vector Concatenate/1, SERIAL_OUT/1
  Vector Concatenate/1 -> PARA_OUT/1

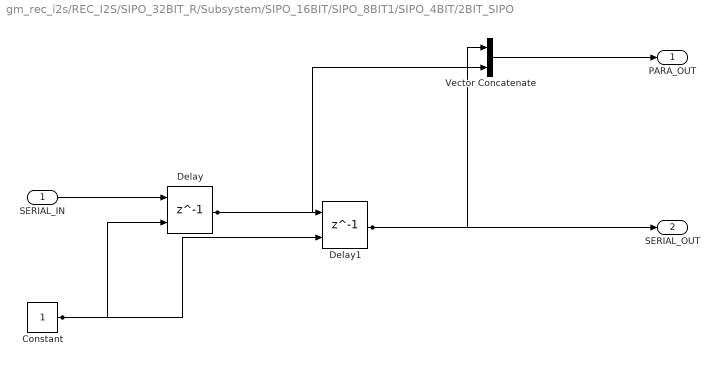
== system gm_rec_i2s/REC_I2S/SIPO_32BIT_R/Subsystem/SIPO_16BIT/SIPO_8BIT1/SIPO_4BIT/2BIT_SIPO ==
  SERIAL_IN : Inport  OutDataTypeStr=boolean  PortDimensions=1  SampleTime=1
  Constant : Constant  OutDataTypeStr=boolean  SampleTime=1
  Delay : Delay  DelayLength=1  InitialCondition=0  ShowEnablePort=on  SampleTime=1
      settings: InputPortMap=u0,e6
  Delay1 : Delay  DelayLength=1  InitialCondition=0  ShowEnablePort=on  SampleTime=1
      settings: InputPortMap=u0,e6
  Vector Concatenate : Concatenate
  PARA_OUT : Outport  SampleTime=1  VectorParamsAs1DForOutWhenUnconnected=off
  SERIAL_OUT : Outport  Port=2  SampleTime=1  VectorParamsAs1DForOutWhenUnconnected=off
  wires:
  SERIAL_IN/1 -> Delay/1
  Constant/1 -> Delay1/2, Delay/2
  Delay/1 -> Vector Concatenate/2, Delay1/1
  Delay1/1 -> Vector Concatenate/1, SERIAL_OUT/1
  Vector Concatenate/1 -> PARA_OUT/1

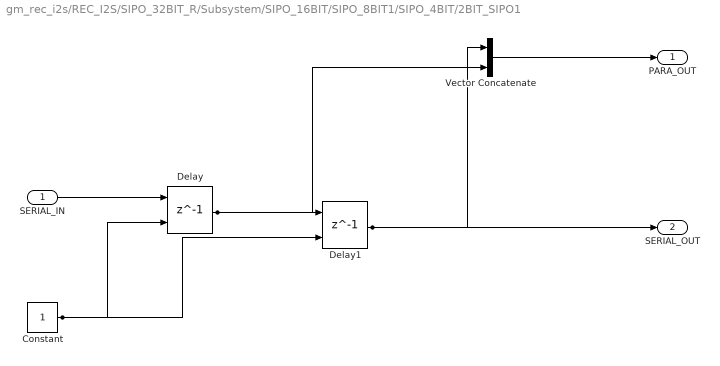
== system gm_rec_i2s/REC_I2S/SIPO_32BIT_R/Subsystem/SIPO_16BIT/SIPO_8BIT1/SIPO_4BIT/2BIT_SIPO1 ==
  SERIAL_IN : Inport  OutDataTypeStr=boolean  PortDimensions=1  SampleTime=1
  Constant : Constant  OutDataTypeStr=boolean  SampleTime=1
  Delay : Delay  DelayLength=1  InitialCondition=0  ShowEnablePort=on  SampleTime=1
      settings: InputPortMap=u0,e6
  Delay1 : Delay  DelayLength=1  InitialCondition=0  ShowEnablePort=on  SampleTime=1
      settings: InputPortMap=u0,e6
  Vector Concatenate : Concatenate
  PARA_OUT : Outport  SampleTime=1  VectorParamsAs1DForOutWhenUnconnected=off
  SERIAL_OUT : Outport  Port=2  SampleTime=1  VectorParamsAs1DForOutWhenUnconnected=off
  wires:
  SERIAL_IN/1 -> Delay/1
  Constant/1 -> Delay1/2, Delay/2
  Delay/1 -> Vector Concatenate/2, Delay1/1
  Delay1/1 -> Vector Concatenate/1, SERIAL_OUT/1
  Vector Concatenate/1 -> PARA_OUT/1

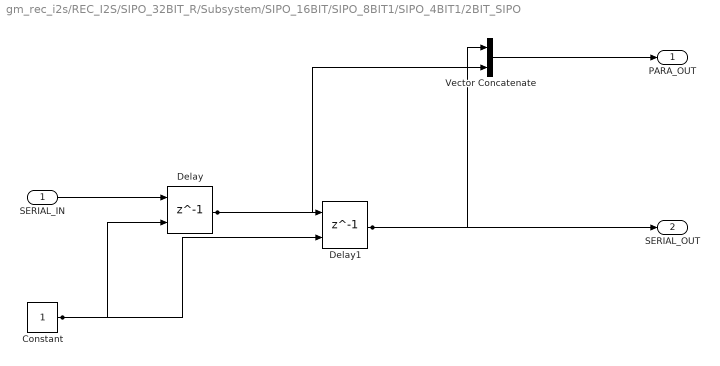
== system gm_rec_i2s/REC_I2S/SIPO_32BIT_R/Subsystem/SIPO_16BIT/SIPO_8BIT1/SIPO_4BIT1/2BIT_SIPO ==
  SERIAL_IN : Inport  OutDataTypeStr=boolean  PortDimensions=1  SampleTime=1
  Constant : Constant  OutDataTypeStr=boolean  SampleTime=1
  Delay : Delay  DelayLength=1  InitialCondition=0  ShowEnablePort=on  SampleTime=1
      settings: InputPortMap=u0,e6
  Delay1 : Delay  DelayLength=1  InitialCondition=0  ShowEnablePort=on  SampleTime=1
      settings: InputPortMap=u0,e6
  Vector Concatenate : Concatenate
  PARA_OUT : Outport  SampleTime=1  VectorParamsAs1DForOutWhenUnconnected=off
  SERIAL_OUT : Outport  Port=2  SampleTime=1  VectorParamsAs1DForOutWhenUnconnected=off
  wires:
  SERIAL_IN/1 -> Delay/1
  Constant/1 -> Delay1/2, Delay/2
  Delay/1 -> Vector Concatenate/2, Delay1/1
  Delay1/1 -> Vector Concatenate/1, SERIAL_OUT/1
  Vector Concatenate/1 -> PARA_OUT/1

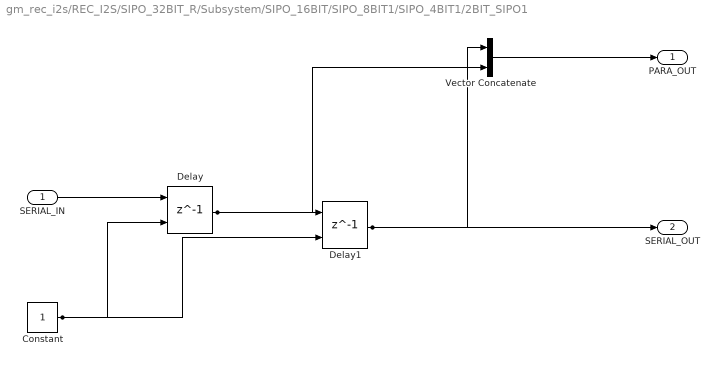
== system gm_rec_i2s/REC_I2S/SIPO_32BIT_R/Subsystem/SIPO_16BIT/SIPO_8BIT1/SIPO_4BIT1/2BIT_SIPO1 ==
  SERIAL_IN : Inport  OutDataTypeStr=boolean  PortDimensions=1  SampleTime=1
  Constant : Constant  OutDataTypeStr=boolean  SampleTime=1
  Delay : Delay  DelayLength=1  InitialCondition=0  ShowEnablePort=on  SampleTime=1
      settings: InputPortMap=u0,e6
  Delay1 : Delay  DelayLength=1  InitialCondition=0  ShowEnablePort=on  SampleTime=1
      settings: InputPortMap=u0,e6
  Vector Concatenate : Concatenate
  PARA_OUT : Outport  SampleTime=1  VectorParamsAs1DForOutWhenUnconnected=off
  SERIAL_OUT : Outport  Port=2  SampleTime=1  VectorParamsAs1DForOutWhenUnconnected=off
  wires:
  SERIAL_IN/1 -> Delay/1
  Constant/1 -> Delay1/2, Delay/2
  Delay/1 -> Vector Concatenate/2, Delay1/1
  Delay1/1 -> Vector Concatenate/1, SERIAL_OUT/1
  Vector Concatenate/1 -> PARA_OUT/1

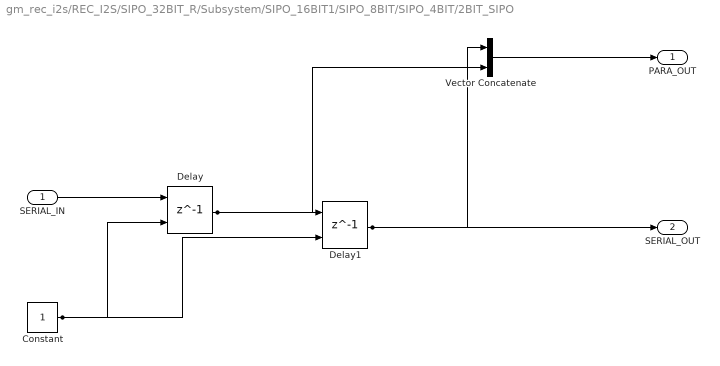
== system gm_rec_i2s/REC_I2S/SIPO_32BIT_R/Subsystem/SIPO_16BIT1/SIPO_8BIT/SIPO_4BIT/2BIT_SIPO ==
  SERIAL_IN : Inport  OutDataTypeStr=boolean  PortDimensions=1  SampleTime=1
  Constant : Constant  OutDataTypeStr=boolean  SampleTime=1
  Delay : Delay  DelayLength=1  InitialCondition=0  ShowEnablePort=on  SampleTime=1
      settings: InputPortMap=u0,e6
  Delay1 : Delay  DelayLength=1  InitialCondition=0  ShowEnablePort=on  SampleTime=1
      settings: InputPortMap=u0,e6
  Vector Concatenate : Concatenate
  PARA_OUT : Outport  SampleTime=1  VectorParamsAs1DForOutWhenUnconnected=off
  SERIAL_OUT : Outport  Port=2  SampleTime=1  VectorParamsAs1DForOutWhenUnconnected=off
  wires:
  SERIAL_IN/1 -> Delay/1
  Constant/1 -> Delay1/2, Delay/2
  Delay/1 -> Vector Concatenate/2, Delay1/1
  Delay1/1 -> Vector Concatenate/1, SERIAL_OUT/1
  Vector Concatenate/1 -> PARA_OUT/1

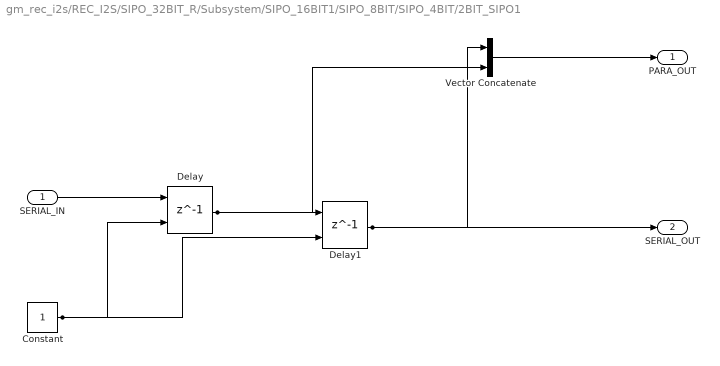
== system gm_rec_i2s/REC_I2S/SIPO_32BIT_R/Subsystem/SIPO_16BIT1/SIPO_8BIT/SIPO_4BIT/2BIT_SIPO1 ==
  SERIAL_IN : Inport  OutDataTypeStr=boolean  PortDimensions=1  SampleTime=1
  Constant : Constant  OutDataTypeStr=boolean  SampleTime=1
  Delay : Delay  DelayLength=1  InitialCondition=0  ShowEnablePort=on  SampleTime=1
      settings: InputPortMap=u0,e6
  Delay1 : Delay  DelayLength=1  InitialCondition=0  ShowEnablePort=on  SampleTime=1
      settings: InputPortMap=u0,e6
  Vector Concatenate : Concatenate
  PARA_OUT : Outport  SampleTime=1  VectorParamsAs1DForOutWhenUnconnected=off
  SERIAL_OUT : Outport  Port=2  SampleTime=1  VectorParamsAs1DForOutWhenUnconnected=off
  wires:
  SERIAL_IN/1 -> Delay/1
  Constant/1 -> Delay1/2, Delay/2
  Delay/1 -> Vector Concatenate/2, Delay1/1
  Delay1/1 -> Vector Concatenate/1, SERIAL_OUT/1
  Vector Concatenate/1 -> PARA_OUT/1

== system gm_rec_i2s/REC_I2S/SIPO_32BIT_R/Subsystem/SIPO_16BIT1/SIPO_8BIT/SIPO_4BIT1/2BIT_SIPO ==
  SERIAL_IN : Inport  OutDataTypeStr=boolean  PortDimensions=1  SampleTime=1
  Constant : Constant  OutDataTypeStr=boolean  SampleTime=1
  Delay : Delay  DelayLength=1  InitialCondition=0  ShowEnablePort=on  SampleTime=1
      settings: InputPortMap=u0,e6
  Delay1 : Delay  DelayLength=1  InitialCondition=0  ShowEnablePort=on  SampleTime=1
      settings: InputPortMap=u0,e6
  Vector Concatenate : Concatenate
  PARA_OUT : Outport  SampleTime=1  VectorParamsAs1DForOutWhenUnconnected=off
  SERIAL_OUT : Outport  Port=2  SampleTime=1  VectorParamsAs1DForOutWhenUnconnected=off
  wires:
  SERIAL_IN/1 -> Delay/1
  Constant/1 -> Delay1/2, Delay/2
  Delay/1 -> Vector Concatenate/2, Delay1/1
  Delay1/1 -> Vector Concatenate/1, SERIAL_OUT/1
  Vector Concatenate/1 -> PARA_OUT/1

== system gm_rec_i2s/REC_I2S/SIPO_32BIT_R/Subsystem/SIPO_16BIT1/SIPO_8BIT/SIPO_4BIT1/2BIT_SIPO1 ==
  SERIAL_IN : Inport  OutDataTypeStr=boolean  PortDimensions=1  SampleTime=1
  Constant : Constant  OutDataTypeStr=boolean  SampleTime=1
  Delay : Delay  DelayLength=1  InitialCondition=0  ShowEnablePort=on  SampleTime=1
      settings: InputPortMap=u0,e6
  Delay1 : Delay  DelayLength=1  InitialCondition=0  ShowEnablePort=on  SampleTime=1
      settings: InputPortMap=u0,e6
  Vector Concatenate : Concatenate
  PARA_OUT : Outport  SampleTime=1  VectorParamsAs1DForOutWhenUnconnected=off
  SERIAL_OUT : Outport  Port=2  SampleTime=1  VectorParamsAs1DForOutWhenUnconnected=off
  wires:
  SERIAL_IN/1 -> Delay/1
  Constant/1 -> Delay1/2, Delay/2
  Delay/1 -> Vector Concatenate/2, Delay1/1
  Delay1/1 -> Vector Concatenate/1, SERIAL_OUT/1
  Vector Concatenate/1 -> PARA_OUT/1

== system gm_rec_i2s/REC_I2S/SIPO_32BIT_R/Subsystem/SIPO_16BIT1/SIPO_8BIT1/SIPO_4BIT/2BIT_SIPO ==
  SERIAL_IN : Inport  OutDataTypeStr=boolean  PortDimensions=1  SampleTime=1
  Constant : Constant  OutDataTypeStr=boolean  SampleTime=1
  Delay : Delay  DelayLength=1  InitialCondition=0  ShowEnablePort=on  SampleTime=1
      settings: InputPortMap=u0,e6
  Delay1 : Delay  DelayLength=1  InitialCondition=0  ShowEnablePort=on  SampleTime=1
      settings: InputPortMap=u0,e6
  Vector Concatenate : Concatenate
  PARA_OUT : Outport  SampleTime=1  VectorParamsAs1DForOutWhenUnconnected=off
  SERIAL_OUT : Outport  Port=2  SampleTime=1  VectorParamsAs1DForOutWhenUnconnected=off
  wires:
  SERIAL_IN/1 -> Delay/1
  Constant/1 -> Delay1/2, Delay/2
  Delay/1 -> Vector Concatenate/2, Delay1/1
  Delay1/1 -> Vector Concatenate/1, SERIAL_OUT/1
  Vector Concatenate/1 -> PARA_OUT/1

== system gm_rec_i2s/REC_I2S/SIPO_32BIT_R/Subsystem/SIPO_16BIT1/SIPO_8BIT1/SIPO_4BIT/2BIT_SIPO1 ==
  SERIAL_IN : Inport  OutDataTypeStr=boolean  PortDimensions=1  SampleTime=1
  Constant : Constant  OutDataTypeStr=boolean  SampleTime=1
  Delay : Delay  DelayLength=1  InitialCondition=0  ShowEnablePort=on  SampleTime=1
      settings: InputPortMap=u0,e6
  Delay1 : Delay  DelayLength=1  InitialCondition=0  ShowEnablePort=on  SampleTime=1
      settings: InputPortMap=u0,e6
  Vector Concatenate : Concatenate
  PARA_OUT : Outport  SampleTime=1  VectorParamsAs1DForOutWhenUnconnected=off
  SERIAL_OUT : Outport  Port=2  SampleTime=1  VectorParamsAs1DForOutWhenUnconnected=off
  wires:
  SERIAL_IN/1 -> Delay/1
  Constant/1 -> Delay1/2, Delay/2
  Delay/1 -> Vector Concatenate/2, Delay1/1
  Delay1/1 -> Vector Concatenate/1, SERIAL_OUT/1
  Vector Concatenate/1 -> PARA_OUT/1

== system gm_rec_i2s/REC_I2S/SIPO_32BIT_R/Subsystem/SIPO_16BIT1/SIPO_8BIT1/SIPO_4BIT1/2BIT_SIPO ==
  SERIAL_IN : Inport  OutDataTypeStr=boolean  PortDimensions=1  SampleTime=1
  Constant : Constant  OutDataTypeStr=boolean  SampleTime=1
  Delay : Delay  DelayLength=1  InitialCondition=0  ShowEnablePort=on  SampleTime=1
      settings: InputPortMap=u0,e6
  Delay1 : Delay  DelayLength=1  InitialCondition=0  ShowEnablePort=on  SampleTime=1
      settings: InputPortMap=u0,e6
  Vector Concatenate : Concatenate
  PARA_OUT : Outport  SampleTime=1  VectorParamsAs1DForOutWhenUnconnected=off
  SERIAL_OUT : Outport  Port=2  SampleTime=1  VectorParamsAs1DForOutWhenUnconnected=off
  wires:
  SERIAL_IN/1 -> Delay/1
  Constant/1 -> Delay1/2, Delay/2
  Delay/1 -> Vector Concatenate/2, Delay1/1
  Delay1/1 -> Vector Concatenate/1, SERIAL_OUT/1
  Vector Concatenate/1 -> PARA_OUT/1

== system gm_rec_i2s/REC_I2S/SIPO_32BIT_R/Subsystem/SIPO_16BIT1/SIPO_8BIT1/SIPO_4BIT1/2BIT_SIPO1 ==
  SERIAL_IN : Inport  OutDataTypeStr=boolean  PortDimensions=1  SampleTime=1
  Constant : Constant  OutDataTypeStr=boolean  SampleTime=1
  Delay : Delay  DelayLength=1  InitialCondition=0  ShowEnablePort=on  SampleTime=1
      settings: InputPortMap=u0,e6
  Delay1 : Delay  DelayLength=1  InitialCondition=0  ShowEnablePort=on  SampleTime=1
      settings: InputPortMap=u0,e6
  Vector Concatenate : Concatenate
  PARA_OUT : Outport  SampleTime=1  VectorParamsAs1DForOutWhenUnconnected=off
  wires:
  SERIAL_IN/1 -> Delay/1
  Constant/1 -> Delay1/2, Delay/2
  Delay/1 -> Vector Concatenate/2, Delay1/1
  Delay1/1 -> Vector Concatenate/1
  Vector Concatenate/1 -> PARA_OUT/1

== system gm_rec_i2s/REC_I2S/SIPO_32BIT_R1/Subsystem/SIPO_16BIT/SIPO_8BIT/SIPO_4BIT/2BIT_SIPO ==
  SERIAL_IN : Inport  OutDataTypeStr=boolean  PortDimensions=1  SampleTime=1
  Constant : Constant  OutDataTypeStr=boolean  SampleTime=1
  Delay : Delay  DelayLength=1  InitialCondition=0  ShowEnablePort=on  SampleTime=1
      settings: InputPortMap=u0,e6
  Delay1 : Delay  DelayLength=1  InitialCondition=0  ShowEnablePort=on  SampleTime=1
      settings: InputPortMap=u0,e6
  Vector Concatenate : Concatenate
  PARA_OUT : Outport  SampleTime=1  VectorParamsAs1DForOutWhenUnconnected=off
  SERIAL_OUT : Outport  Port=2  SampleTime=1  VectorParamsAs1DForOutWhenUnconnected=off
  wires:
  SERIAL_IN/1 -> Delay/1
  Constant/1 -> Delay1/2, Delay/2
  Delay/1 -> Vector Concatenate/2, Delay1/1
  Delay1/1 -> Vector Concatenate/1, SERIAL_OUT/1
  Vector Concatenate/1 -> PARA_OUT/1

== system gm_rec_i2s/REC_I2S/SIPO_32BIT_R1/Subsystem/SIPO_16BIT/SIPO_8BIT/SIPO_4BIT/2BIT_SIPO1 ==
  SERIAL_IN : Inport  OutDataTypeStr=boolean  PortDimensions=1  SampleTime=1
  Constant : Constant  OutDataTypeStr=boolean  SampleTime=1
  Delay : Delay  DelayLength=1  InitialCondition=0  ShowEnablePort=on  SampleTime=1
      settings: InputPortMap=u0,e6
  Delay1 : Delay  DelayLength=1  InitialCondition=0  ShowEnablePort=on  SampleTime=1
      settings: InputPortMap=u0,e6
  Vector Concatenate : Concatenate
  PARA_OUT : Outport  SampleTime=1  VectorParamsAs1DForOutWhenUnconnected=off
  SERIAL_OUT : Outport  Port=2  SampleTime=1  VectorParamsAs1DForOutWhenUnconnected=off
  wires:
  SERIAL_IN/1 -> Delay/1
  Constant/1 -> Delay1/2, Delay/2
  Delay/1 -> Vector Concatenate/2, Delay1/1
  Delay1/1 -> Vector Concatenate/1, SERIAL_OUT/1
  Vector Concatenate/1 -> PARA_OUT/1

== system gm_rec_i2s/REC_I2S/SIPO_32BIT_R1/Subsystem/SIPO_16BIT/SIPO_8BIT/SIPO_4BIT1/2BIT_SIPO ==
  SERIAL_IN : Inport  OutDataTypeStr=boolean  PortDimensions=1  SampleTime=1
  Constant : Constant  OutDataTypeStr=boolean  SampleTime=1
  Delay : Delay  DelayLength=1  InitialCondition=0  ShowEnablePort=on  SampleTime=1
      settings: InputPortMap=u0,e6
  Delay1 : Delay  DelayLength=1  InitialCondition=0  ShowEnablePort=on  SampleTime=1
      settings: InputPortMap=u0,e6
  Vector Concatenate : Concatenate
  PARA_OUT : Outport  SampleTime=1  VectorParamsAs1DForOutWhenUnconnected=off
  SERIAL_OUT : Outport  Port=2  SampleTime=1  VectorParamsAs1DForOutWhenUnconnected=off
  wires:
  SERIAL_IN/1 -> Delay/1
  Constant/1 -> Delay1/2, Delay/2
  Delay/1 -> Vector Concatenate/2, Delay1/1
  Delay1/1 -> Vector Concatenate/1, SERIAL_OUT/1
  Vector Concatenate/1 -> PARA_OUT/1

== system gm_rec_i2s/REC_I2S/SIPO_32BIT_R1/Subsystem/SIPO_16BIT/SIPO_8BIT/SIPO_4BIT1/2BIT_SIPO1 ==
  SERIAL_IN : Inport  OutDataTypeStr=boolean  PortDimensions=1  SampleTime=1
  Constant : Constant  OutDataTypeStr=boolean  SampleTime=1
  Delay : Delay  DelayLength=1  InitialCondition=0  ShowEnablePort=on  SampleTime=1
      settings: InputPortMap=u0,e6
  Delay1 : Delay  DelayLength=1  InitialCondition=0  ShowEnablePort=on  SampleTime=1
      settings: InputPortMap=u0,e6
  Vector Concatenate : Concatenate
  PARA_OUT : Outport  SampleTime=1  VectorParamsAs1DForOutWhenUnconnected=off
  SERIAL_OUT : Outport  Port=2  SampleTime=1  VectorParamsAs1DForOutWhenUnconnected=off
  wires:
  SERIAL_IN/1 -> Delay/1
  Constant/1 -> Delay1/2, Delay/2
  Delay/1 -> Vector Concatenate/2, Delay1/1
  Delay1/1 -> Vector Concatenate/1, SERIAL_OUT/1
  Vector Concatenate/1 -> PARA_OUT/1

== system gm_rec_i2s/REC_I2S/SIPO_32BIT_R1/Subsystem/SIPO_16BIT/SIPO_8BIT1/SIPO_4BIT/2BIT_SIPO ==
  SERIAL_IN : Inport  OutDataTypeStr=boolean  PortDimensions=1  SampleTime=1
  Constant : Constant  OutDataTypeStr=boolean  SampleTime=1
  Delay : Delay  DelayLength=1  InitialCondition=0  ShowEnablePort=on  SampleTime=1
      settings: InputPortMap=u0,e6
  Delay1 : Delay  DelayLength=1  InitialCondition=0  ShowEnablePort=on  SampleTime=1
      settings: InputPortMap=u0,e6
  Vector Concatenate : Concatenate
  PARA_OUT : Outport  SampleTime=1  VectorParamsAs1DForOutWhenUnconnected=off
  SERIAL_OUT : Outport  Port=2  SampleTime=1  VectorParamsAs1DForOutWhenUnconnected=off
  wires:
  SERIAL_IN/1 -> Delay/1
  Constant/1 -> Delay1/2, Delay/2
  Delay/1 -> Vector Concatenate/2, Delay1/1
  Delay1/1 -> Vector Concatenate/1, SERIAL_OUT/1
  Vector Concatenate/1 -> PARA_OUT/1

== system gm_rec_i2s/REC_I2S/SIPO_32BIT_R1/Subsystem/SIPO_16BIT/SIPO_8BIT1/SIPO_4BIT/2BIT_SIPO1 ==
  SERIAL_IN : Inport  OutDataTypeStr=boolean  PortDimensions=1  SampleTime=1
  Constant : Constant  OutDataTypeStr=boolean  SampleTime=1
  Delay : Delay  DelayLength=1  InitialCondition=0  ShowEnablePort=on  SampleTime=1
      settings: InputPortMap=u0,e6
  Delay1 : Delay  DelayLength=1  InitialCondition=0  ShowEnablePort=on  SampleTime=1
      settings: InputPortMap=u0,e6
  Vector Concatenate : Concatenate
  PARA_OUT : Outport  SampleTime=1  VectorParamsAs1DForOutWhenUnconnected=off
  SERIAL_OUT : Outport  Port=2  SampleTime=1  VectorParamsAs1DForOutWhenUnconnected=off
  wires:
  SERIAL_IN/1 -> Delay/1
  Constant/1 -> Delay1/2, Delay/2
  Delay/1 -> Vector Concatenate/2, Delay1/1
  Delay1/1 -> Vector Concatenate/1, SERIAL_OUT/1
  Vector Concatenate/1 -> PARA_OUT/1

== system gm_rec_i2s/REC_I2S/SIPO_32BIT_R1/Subsystem/SIPO_16BIT/SIPO_8BIT1/SIPO_4BIT1/2BIT_SIPO ==
  SERIAL_IN : Inport  OutDataTypeStr=boolean  PortDimensions=1  SampleTime=1
  Constant : Constant  OutDataTypeStr=boolean  SampleTime=1
  Delay : Delay  DelayLength=1  InitialCondition=0  ShowEnablePort=on  SampleTime=1
      settings: InputPortMap=u0,e6
  Delay1 : Delay  DelayLength=1  InitialCondition=0  ShowEnablePort=on  SampleTime=1
      settings: InputPortMap=u0,e6
  Vector Concatenate : Concatenate
  PARA_OUT : Outport  SampleTime=1  VectorParamsAs1DForOutWhenUnconnected=off
  SERIAL_OUT : Outport  Port=2  SampleTime=1  VectorParamsAs1DForOutWhenUnconnected=off
  wires:
  SERIAL_IN/1 -> Delay/1
  Constant/1 -> Delay1/2, Delay/2
  Delay/1 -> Vector Concatenate/2, Delay1/1
  Delay1/1 -> Vector Concatenate/1, SERIAL_OUT/1
  Vector Concatenate/1 -> PARA_OUT/1

== system gm_rec_i2s/REC_I2S/SIPO_32BIT_R1/Subsystem/SIPO_16BIT/SIPO_8BIT1/SIPO_4BIT1/2BIT_SIPO1 ==
  SERIAL_IN : Inport  OutDataTypeStr=boolean  PortDimensions=1  SampleTime=1
  Constant : Constant  OutDataTypeStr=boolean  SampleTime=1
  Delay : Delay  DelayLength=1  InitialCondition=0  ShowEnablePort=on  SampleTime=1
      settings: InputPortMap=u0,e6
  Delay1 : Delay  DelayLength=1  InitialCondition=0  ShowEnablePort=on  SampleTime=1
      settings: InputPortMap=u0,e6
  Vector Concatenate : Concatenate
  PARA_OUT : Outport  SampleTime=1  VectorParamsAs1DForOutWhenUnconnected=off
  SERIAL_OUT : Outport  Port=2  SampleTime=1  VectorParamsAs1DForOutWhenUnconnected=off
  wires:
  SERIAL_IN/1 -> Delay/1
  Constant/1 -> Delay1/2, Delay/2
  Delay/1 -> Vector Concatenate/2, Delay1/1
  Delay1/1 -> Vector Concatenate/1, SERIAL_OUT/1
  Vector Concatenate/1 -> PARA_OUT/1

== system gm_rec_i2s/REC_I2S/SIPO_32BIT_R1/Subsystem/SIPO_16BIT1/SIPO_8BIT/SIPO_4BIT/2BIT_SIPO ==
  SERIAL_IN : Inport  OutDataTypeStr=boolean  PortDimensions=1  SampleTime=1
  Constant : Constant  OutDataTypeStr=boolean  SampleTime=1
  Delay : Delay  DelayLength=1  InitialCondition=0  ShowEnablePort=on  SampleTime=1
      settings: InputPortMap=u0,e6
  Delay1 : Delay  DelayLength=1  InitialCondition=0  ShowEnablePort=on  SampleTime=1
      settings: InputPortMap=u0,e6
  Vector Concatenate : Concatenate
  PARA_OUT : Outport  SampleTime=1  VectorParamsAs1DForOutWhenUnconnected=off
  SERIAL_OUT : Outport  Port=2  SampleTime=1  VectorParamsAs1DForOutWhenUnconnected=off
  wires:
  SERIAL_IN/1 -> Delay/1
  Constant/1 -> Delay1/2, Delay/2
  Delay/1 -> Vector Concatenate/2, Delay1/1
  Delay1/1 -> Vector Concatenate/1, SERIAL_OUT/1
  Vector Concatenate/1 -> PARA_OUT/1

== system gm_rec_i2s/REC_I2S/SIPO_32BIT_R1/Subsystem/SIPO_16BIT1/SIPO_8BIT/SIPO_4BIT/2BIT_SIPO1 ==
  SERIAL_IN : Inport  OutDataTypeStr=boolean  PortDimensions=1  SampleTime=1
  Constant : Constant  OutDataTypeStr=boolean  SampleTime=1
  Delay : Delay  DelayLength=1  InitialCondition=0  ShowEnablePort=on  SampleTime=1
      settings: InputPortMap=u0,e6
  Delay1 : Delay  DelayLength=1  InitialCondition=0  ShowEnablePort=on  SampleTime=1
      settings: InputPortMap=u0,e6
  Vector Concatenate : Concatenate
  PARA_OUT : Outport  SampleTime=1  VectorParamsAs1DForOutWhenUnconnected=off
  SERIAL_OUT : Outport  Port=2  SampleTime=1  VectorParamsAs1DForOutWhenUnconnected=off
  wires:
  SERIAL_IN/1 -> Delay/1
  Constant/1 -> Delay1/2, Delay/2
  Delay/1 -> Vector Concatenate/2, Delay1/1
  Delay1/1 -> Vector Concatenate/1, SERIAL_OUT/1
  Vector Concatenate/1 -> PARA_OUT/1

== system gm_rec_i2s/REC_I2S/SIPO_32BIT_R1/Subsystem/SIPO_16BIT1/SIPO_8BIT/SIPO_4BIT1/2BIT_SIPO ==
  SERIAL_IN : Inport  OutDataTypeStr=boolean  PortDimensions=1  SampleTime=1
  Constant : Constant  OutDataTypeStr=boolean  SampleTime=1
  Delay : Delay  DelayLength=1  InitialCondition=0  ShowEnablePort=on  SampleTime=1
      settings: InputPortMap=u0,e6
  Delay1 : Delay  DelayLength=1  InitialCondition=0  ShowEnablePort=on  SampleTime=1
      settings: InputPortMap=u0,e6
  Vector Concatenate : Concatenate
  PARA_OUT : Outport  SampleTime=1  VectorParamsAs1DForOutWhenUnconnected=off
  SERIAL_OUT : Outport  Port=2  SampleTime=1  VectorParamsAs1DForOutWhenUnconnected=off
  wires:
  SERIAL_IN/1 -> Delay/1
  Constant/1 -> Delay1/2, Delay/2
  Delay/1 -> Vector Concatenate/2, Delay1/1
  Delay1/1 -> Vector Concatenate/1, SERIAL_OUT/1
  Vector Concatenate/1 -> PARA_OUT/1

== system gm_rec_i2s/REC_I2S/SIPO_32BIT_R1/Subsystem/SIPO_16BIT1/SIPO_8BIT/SIPO_4BIT1/2BIT_SIPO1 ==
  SERIAL_IN : Inport  OutDataTypeStr=boolean  PortDimensions=1  SampleTime=1
  Constant : Constant  OutDataTypeStr=boolean  SampleTime=1
  Delay : Delay  DelayLength=1  InitialCondition=0  ShowEnablePort=on  SampleTime=1
      settings: InputPortMap=u0,e6
  Delay1 : Delay  DelayLength=1  InitialCondition=0  ShowEnablePort=on  SampleTime=1
      settings: InputPortMap=u0,e6
  Vector Concatenate : Concatenate
  PARA_OUT : Outport  SampleTime=1  VectorParamsAs1DForOutWhenUnconnected=off
  SERIAL_OUT : Outport  Port=2  SampleTime=1  VectorParamsAs1DForOutWhenUnconnected=off
  wires:
  SERIAL_IN/1 -> Delay/1
  Constant/1 -> Delay1/2, Delay/2
  Delay/1 -> Vector Concatenate/2, Delay1/1
  Delay1/1 -> Vector Concatenate/1, SERIAL_OUT/1
  Vector Concatenate/1 -> PARA_OUT/1

== system gm_rec_i2s/REC_I2S/SIPO_32BIT_R1/Subsystem/SIPO_16BIT1/SIPO_8BIT1/SIPO_4BIT/2BIT_SIPO ==
  SERIAL_IN : Inport  OutDataTypeStr=boolean  PortDimensions=1  SampleTime=1
  Constant : Constant  OutDataTypeStr=boolean  SampleTime=1
  Delay : Delay  DelayLength=1  InitialCondition=0  ShowEnablePort=on  SampleTime=1
      settings: InputPortMap=u0,e6
  Delay1 : Delay  DelayLength=1  InitialCondition=0  ShowEnablePort=on  SampleTime=1
      settings: InputPortMap=u0,e6
  Vector Concatenate : Concatenate
  PARA_OUT : Outport  SampleTime=1  VectorParamsAs1DForOutWhenUnconnected=off
  SERIAL_OUT : Outport  Port=2  SampleTime=1  VectorParamsAs1DForOutWhenUnconnected=off
  wires:
  SERIAL_IN/1 -> Delay/1
  Constant/1 -> Delay1/2, Delay/2
  Delay/1 -> Vector Concatenate/2, Delay1/1
  Delay1/1 -> Vector Concatenate/1, SERIAL_OUT/1
  Vector Concatenate/1 -> PARA_OUT/1

== system gm_rec_i2s/REC_I2S/SIPO_32BIT_R1/Subsystem/SIPO_16BIT1/SIPO_8BIT1/SIPO_4BIT/2BIT_SIPO1 ==
  SERIAL_IN : Inport  OutDataTypeStr=boolean  PortDimensions=1  SampleTime=1
  Constant : Constant  OutDataTypeStr=boolean  SampleTime=1
  Delay : Delay  DelayLength=1  InitialCondition=0  ShowEnablePort=on  SampleTime=1
      settings: InputPortMap=u0,e6
  Delay1 : Delay  DelayLength=1  InitialCondition=0  ShowEnablePort=on  SampleTime=1
      settings: InputPortMap=u0,e6
  Vector Concatenate : Concatenate
  PARA_OUT : Outport  SampleTime=1  VectorParamsAs1DForOutWhenUnconnected=off
  SERIAL_OUT : Outport  Port=2  SampleTime=1  VectorParamsAs1DForOutWhenUnconnected=off
  wires:
  SERIAL_IN/1 -> Delay/1
  Constant/1 -> Delay1/2, Delay/2
  Delay/1 -> Vector Concatenate/2, Delay1/1
  Delay1/1 -> Vector Concatenate/1, SERIAL_OUT/1
  Vector Concatenate/1 -> PARA_OUT/1
